simulink model "mdl_PI_anti_windup_2"  (R2022b)
settings: Solver=VariableStepAuto  StartTime=0.0  StopTime=0.4  FixedStep=0.001  RelTol=1e-3
settings Model: Creator=jack  LastModifiedBy=jackyeh

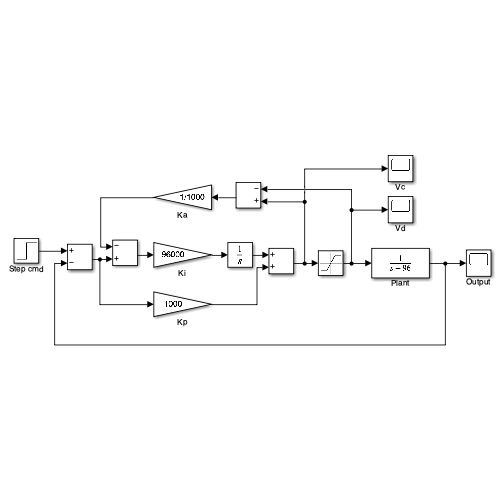
[thumbnail: Simulink's stored preview of the top-level diagram]
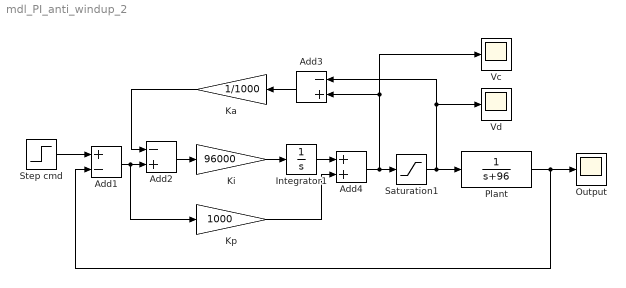
== system mdl_PI_anti_windup_2 ==
  Add1 : Sum  Inputs=+-
  Add2 : Sum  Inputs=-+
  Add3 : Sum  Inputs=-+
  Add4 : Sum
  Integrator1 : Integrator
  Ka : Gain  Gain=1/1000
  Ki : Gain  Gain=96000
  Kp : Gain  Gain=1000
  Output : Scope
  Plant : TransferFcn  Denominator=[1 96]
  Saturation1 : Saturate  UpperLimit=50  LowerLimit=-50
  Step cmd : Step  Time=0.1  SampleTime=0
  Vc : Scope
  Vd : Scope
  wires:
  Step cmd/1 -> Add1/1
  Plant/1 -> Output/1, Add1/2
  Saturation1/1 -> Add3/1, Vd/1, Plant/1
  Add1/1 -> Kp/1, Add2/2
  Add2/1 -> Ki/1
  Ki/1 -> Integrator1/1
  Integrator1/1 -> Add4/1
  Kp/1 -> Add4/2
  Add4/1 -> Vc/1, Add3/2, Saturation1/1
  Add3/1 -> Ka/1
  Ka/1 -> Add2/1
